simulink model "Vehicle_Model_2Track"  (R2021a)
settings: Solver=FixedStepDiscrete  StartTime=T0  StopTime=Tf  FixedStep=Ts  EnableMultiTasking=on
model workspace (MAT data in the model file):
  aKalman = Simulink.Parameter
  aKalman.DataType = 'auto'
  aKalman.Dimensions = [0 0]
  slipEnabler = Simulink.Parameter
  slipEnabler.DataType = 'auto'
  slipEnabler.Dimensions = [0 0]
values from neighbouring files (symbols this model uses):
  pacejkaParam = loadPacejkaParam()    [mainVehicleModel_2Track.m]
  vehicle_data = getVehicleDataStruct()    [mainVehicleModel_2Track.m]
  X0 = loadInitialConditions    [mainVehicleModel_2Track.m]
undefined symbols (not defined in the file or in its folder): DiscIntNeverNeededParam
libraries: simulink_extras x11
settings Model: Creator=Edoardo  LastModifiedBy=basemprince
settings SolverCC: AlgebraicLoopSolver=TrustRegion
settings DataIOCC: LimitDataPoints=on  SaveFormat=Array
settings OptimizationCC: DefaultParameterBehavior=Inlined  PassReuseOutputArgsAs=Individual arguments  MaxStackSize=64  EfficientTunableParamExpr=on
settings DebuggingCC: ReadBeforeWriteMsg=DisableAll  WriteAfterWriteMsg=DisableAll  WriteAfterReadMsg=DisableAll  MultiTaskDSMMsg=none  ParameterTunabilityLossMsg=error  PregeneratedLibrarySubsystemCodeDiagnostic=none  SFUnexpectedBacktrackingDiag=warning  SFNoUnconditionalDefaultTransitionDiag=warning  SFExecutionAtInitializationDiag=none  SFMachineParentedDataDiag=warning  ArithmeticOperatorsInVariantConditions=warning
settings HardwareCC: ProdBitPerInt=16  ProdBitPerPointer=16  ProdBitPerSizeT=16  ProdBitPerPtrDiffT=16  ProdLargestAtomicFloat=None  ProdWordSize=16  ProdHWDeviceType=STMicroelectronics->ST10/Super10
settings ModelReferenceCC: UpdateModelReferenceTargets=IfOutOfDate  PropagateSignalLabelsOutOfModel=off
settings SFSimCC: SFSimEcho=off  SimUseLocalCustomCode=off  MATLABDynamicMemAlloc=off  CustomCodeUndefinedFunction=UseInterfaceOnly
settings RTWCC: SystemTargetFile=ert.tlc  TemplateMakefile=ert_default_tmf  GenerateReport=on  RetainRTWFile=on  RTWUseLocalCustomCode=off  Toolchain=GNU Tools for ARM Embedded Processors  BuildConfiguration=Faster Runs  IncludeHyperlinkInReport=on  LaunchReport=on  GenerateTraceInfo=on  GenerateTraceReport=on  GenerateTraceReportSl=on  GenerateTraceReportSf=on  GenerateTraceReportEml=on
settings CodeAppCC: ForceParamTrailComments=on  IgnoreCustomStorageClasses=off  OperatorAnnotations=on  SimulinkDataObjDesc=on  SFDataObjDesc=on  InsertBlockDesc=on
settings ERTTargetCC: CodeReplacementLibrary=ARM Cortex-M (Optimized)  SupportVariableSizeSignals=on  RootIOFormat=Structure reference  ERTCustomFileTemplate=example_file_process.tlc
settings ConfigComp: CovMetricSettings=dw  CovSaveCumulativeToWorkspaceVar=on  CovSaveSingleToWorkspaceVar=on  CovExternalEMLEnable=off

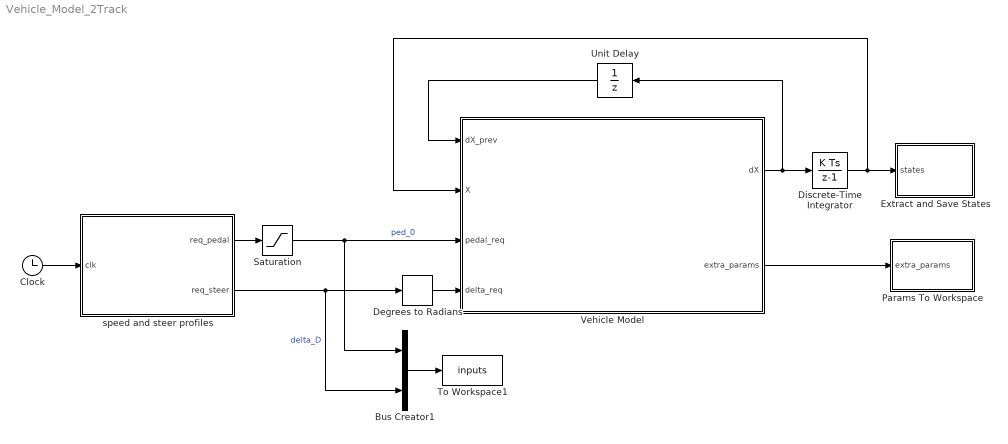
== system Vehicle_Model_2Track ==
  Bus Creator1 : BusCreator  Inputs=2
  Clock : Clock
  Degrees to Radians : simulink_extras/Transformations/Degrees to Radians
  Discrete-Time Integrator : DiscreteIntegrator  gainval=1  InitialCondition=X0  SampleTime=-1  ICPrevOutput=DiscIntNeverNeededParam  ICPrevScaledInput=DiscIntNeverNeededParam
  Extract and Save States : Subsystem
  Params To Workspace : Subsystem
  Saturation : Saturate  UpperLimit=1  LowerLimit=-1
  To Workspace1 : ToWorkspace  VariableName=inputs  SaveFormat=Timeseries  SampleTime=-1
  Unit Delay : UnitDelay  InitialCondition=zeros(size(X0))  SampleTime=-1  HasFrameUpgradeWarning=on
  Vehicle Model : MATLAB Function  TreatAsAtomicUnit=on
  speed and steer profiles : MATLAB Function  TreatAsAtomicUnit=on
  wires:
  Vehicle Model/2(extra_params) -> Params To Workspace/1(extra_params)
  Discrete-Time Integrator/1 -> Extract and Save States/1(states), Vehicle Model/2(X)
  Vehicle Model/1(dX) -> Unit Delay/1, Discrete-Time Integrator/1
  Bus Creator1/1 -> To Workspace1/1
  speed and steer profiles/2(req_steer) -> Bus Creator1/2, Degrees to Radians/1  "delta_D"
  Degrees to Radians/1 -> Vehicle Model/4(delta_req)
  speed and steer profiles/1(req_pedal) -> Saturation/1
  Clock/1 -> speed and steer profiles/1(clk)
  Saturation/1 -> Vehicle Model/3(pedal_req), Bus Creator1/1  "ped_0"
  Unit Delay/1 -> Vehicle Model/1(dX_prev)

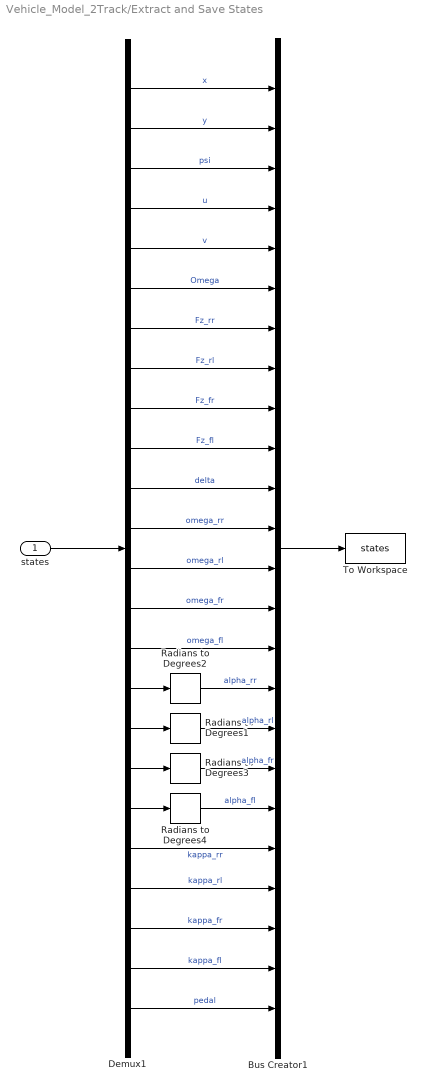
== system Vehicle_Model_2Track/Extract and Save States ==
  states : Inport
  Bus Creator1 : BusCreator  Inputs=24
  Demux1 : Demux  Outputs=24
  Radians to Degrees{1..4} (4 alike) : simulink_extras/Transformations/Radians to Degrees
  To Workspace : ToWorkspace  VariableName=states  SaveFormat=Timeseries  SampleTime=-1
  wires:
  Demux1/13 -> Bus Creator1/13  "omega_rl"
  Demux1/8 -> Bus Creator1/8  "Fz_rl"
  Demux1/23 -> Bus Creator1/23  "kappa_fl"
  Demux1/19 -> Radians to Degrees4/1
  states/1 -> Demux1/1
  Demux1/14 -> Bus Creator1/14  "omega_fr"
  Demux1/7 -> Bus Creator1/7  "Fz_rr"
  Demux1/15 -> Bus Creator1/15  "omega_fl"
  Demux1/3 -> Bus Creator1/3  "psi"
  Demux1/22 -> Bus Creator1/22  "kappa_fr"
  Demux1/4 -> Bus Creator1/4  "u"
  Demux1/6 -> Bus Creator1/6  "Omega"
  Demux1/11 -> Bus Creator1/11  "delta"
  Demux1/5 -> Bus Creator1/5  "v"
  Demux1/9 -> Bus Creator1/9  "Fz_fr"
  Demux1/21 -> Bus Creator1/21  "kappa_rl"
  Demux1/12 -> Bus Creator1/12  "omega_rr"
  Demux1/17 -> Radians to Degrees1/1
  Demux1/2 -> Bus Creator1/2  "y"
  Demux1/20 -> Bus Creator1/20  "kappa_rr"
  Demux1/10 -> Bus Creator1/10  "Fz_fl"
  Demux1/18 -> Radians to Degrees3/1
  Demux1/1 -> Bus Creator1/1  "x"
  Demux1/16 -> Radians to Degrees2/1
  Bus Creator1/1 -> To Workspace/1
  Radians to Degrees2/1 -> Bus Creator1/16  "alpha_rr"
  Radians to Degrees1/1 -> Bus Creator1/17  "alpha_rl"
  Radians to Degrees3/1 -> Bus Creator1/18  "alpha_fr"
  Radians to Degrees4/1 -> Bus Creator1/19  "alpha_fl"
  Demux1/24 -> Bus Creator1/24  "pedal"

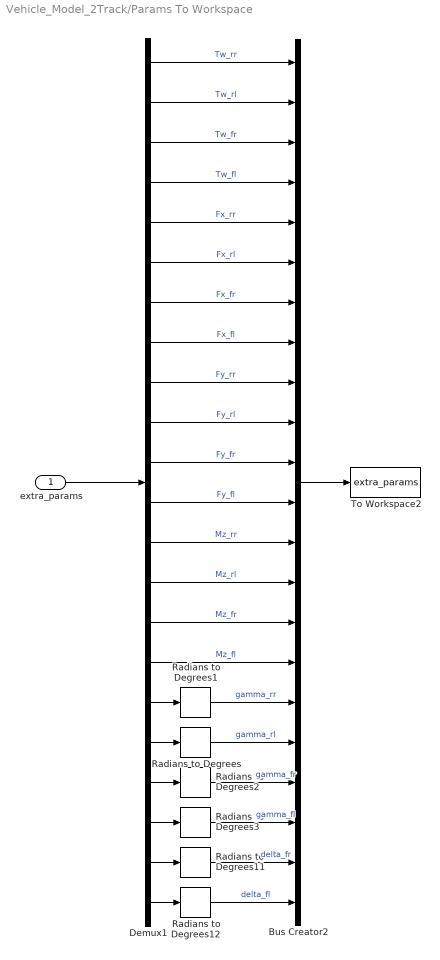
== system Vehicle_Model_2Track/Params To Workspace ==
  extra_params : Inport
  Bus Creator2 : BusCreator  Inputs=22
  Demux1 : Demux  Outputs=22
  Radians to Degrees{,1..3,11..12} (6 alike) : simulink_extras/Transformations/Radians to Degrees
  To Workspace2 : ToWorkspace  VariableName=extra_params  SaveFormat=Timeseries  SampleTime=-1
  wires:
  Demux1/17 -> Radians to Degrees1/1
  Demux1/3 -> Bus Creator2/3  "Tw_fr"
  Radians to Degrees3/1 -> Bus Creator2/20  "gamma_fl"
  Demux1/16 -> Bus Creator2/16  "Mz_fl"
  Radians to Degrees1/1 -> Bus Creator2/17  "gamma_rr"
  Radians to Degrees11/1 -> Bus Creator2/21  "delta_fr"
  Demux1/14 -> Bus Creator2/14  "Mz_rl"
  Demux1/4 -> Bus Creator2/4  "Tw_fl"
  Demux1/6 -> Bus Creator2/6  "Fx_rl"
  Demux1/8 -> Bus Creator2/8  "Fx_fl"
  Demux1/13 -> Bus Creator2/13  "Mz_rr"
  Demux1/7 -> Bus Creator2/7  "Fx_fr"
  Demux1/5 -> Bus Creator2/5  "Fx_rr"
  Demux1/9 -> Bus Creator2/9  "Fy_rr"
  Demux1/11 -> Bus Creator2/11  "Fy_fr"
  Demux1/15 -> Bus Creator2/15  "Mz_fr"
  Demux1/10 -> Bus Creator2/10  "Fy_rl"
  Radians to Degrees12/1 -> Bus Creator2/22  "delta_fl"
  Radians to Degrees2/1 -> Bus Creator2/19  "gamma_fr"
  extra_params/1 -> Demux1/1
  Demux1/12 -> Bus Creator2/12  "Fy_fl"
  Bus Creator2/1 -> To Workspace2/1
  Demux1/1 -> Bus Creator2/1  "Tw_rr"
  Demux1/2 -> Bus Creator2/2  "Tw_rl"
  Radians to Degrees/1 -> Bus Creator2/18  "gamma_rl"
  Demux1/18 -> Radians to Degrees/1
  Demux1/19 -> Radians to Degrees2/1
  Demux1/20 -> Radians to Degrees3/1
  Demux1/21 -> Radians to Degrees11/1
  Demux1/22 -> Radians to Degrees12/1

== matlab function Vehicle_Model_2Track/speed and steer profiles ==
  data: clk input; req_pedal output; req_steer output
function [req_pedal,req_steer] = pedal_steer_profiles(clk)

    % ----------------------------------------------------------------
    %% Function purpose: compute the desired pedal and steer profiles
    % ----------------------------------------------------------------
    
    % Requested pedal [-] in [-1,1] for this time step.
    % req_pedal > 0 means throttle
    % req_pedal < 0 means brake
    req_pedal = -0.5;
    
    % Requested steering angle [deg] at the steering wheel for this time step
    req_steer = 1*sin(2*pi*0.18*clk);

end

== matlab function Vehicle_Model_2Track/Vehicle Model ==
  settings: sampleTime=step_size
  data: dX_prev input; X input; dX output; extra_params output; pedal_req input; delta_req input; pacejkaParam parameter; vehicle_data parameter
function [dX,extra_params] = Vehicle_model(dX_prev,X,pedal_req,delta_req,pacejkaParam,vehicle_data)

% ----------------------------------------------------------------
%% Double Track Vehicle Model of Formula SAE electric vehicle (Chimera Evoluzione)
%  authors: Mattia Piccinini & Gastone Pietro Papini Rosati
%  email:  mattia.piccinini@unitn.it
%  date:   13/10/2020
% ----------------------------------------------------------------


% ----------------------------------------------------------------
%% INPUTS OF THE MODEL
% ----------------------------------------------------------------

% Model inputs are: 
%       - requested pedal (throttle if >0, brake if <0)
%       - requested steering angle at the steering wheel delta_req (in [rad])


% ----------------------------------------------------------------
%% OUTPUTS OF THE MODEL
% ----------------------------------------------------------------

% The outputs of the model are the derivatives of all vehicle states,
% collected in the dX vector, as well as some other useful extra parameters 
% to describe vehicle behavior, saved in the extra_params vector

% Empty output vectors are here initialized 
dX = zeros(24,1);  
extra_params = zeros(22,1);  


% ----------------------------------------------------------------
%% STATES OF THE MODEL
% ----------------------------------------------------------------

x         = X(1);       % [m] x-coord of the vehicle CoM
y         = X(2);       % [m] y-coord of the vehicle CoM
psi       = X(3);       % [rad] yaw angle
u         = X(4);       % [m/s] vehicle longitudinal speed
v         = X(5);       % [m/s] vehicle lateral speed
Omega     = X(6);       % [rad/s] yaw rate
Fz__rr    = X(7);       % [N] vertical force for the rear right wheel
Fz__rl    = X(8);       % [N] vertical force for the rear left wheel
Fz__fr    = X(9);       % [N] vertical force for the front right wheel
Fz__fl    = X(10);      % [N] vertical force for the front left wheel
delta     = X(11);      % [rad] steering angle (at the wheel)
omega__rr = X(12);      % [rad/s] rotational speed rear right wheel
omega__rl = X(13);      % [rad/s] rotational speed rear left wheel 
omega__fr = X(14);      % [rad/s] rotational speed front right wheel 
omega__fl = X(15);      % [rad/s] rotational speed front left wheel 
alpha__rr = X(16);      % [rad] side slip angle rear right wheel
alpha__rl = X(17);      % [rad] side slip angle rear left wheel
alpha__fr = X(18);      % [rad] side slip angle front right wheel
alpha__fl = X(19);      % [rad] side slip angle front left wheel
kappa__rr = X(20);      % [-] longitudinal slip rear right wheel
kappa__rl = X(21);      % [-] longitudinal slip rear left wheel
kappa__fr = X(22);      % [-] longitudinal slip front right wheel
kappa__fl = X(23);      % [-] longitudinal slip front left wheel
ped       = X(24);      % [-] pedal

% ----------------------------------------------------------------
%% AUXILIARY MODELS
% ----------------------------------------------------------------

% ----------------------
% MOTOR MODEL
% ----------------------
% Driving torques at the wheels
Tm_req = posPart(ped)*vehicle_data.motor.maxTorque;
Tw__rr_traction = MotorModel(Tm_req,omega__rr,vehicle_data);
Tw__rl_traction = MotorModel(Tm_req,omega__rl,vehicle_data);
 
% ----------------------
% BRAKE MODEL
% ----------------------
Tb_r_req = -negPart(ped)*vehicle_data.braking.totBrakeTorque*(1-vehicle_data.braking.brakeRatio);
Tb_f_req = -negPart(ped)*vehicle_data.braking.totBrakeTorque*vehicle_data.braking.brakeRatio;
% Rear wheels braking model
[Tw__rr_brake,Tw__rl_brake] = brakeModelRear(Tb_r_req,omega__rr,omega__rl,vehicle_data); 
% Front wheels braking model
[Tw__fr_brake,Tw__fl_brake] = brakeModelFront(Tb_f_req,omega__fr,omega__fl,vehicle_data);

% ----------------------
% WHEEL TORQUES
% ----------------------
% The total torque for each wheel is the algebraic sum of motor and brake torques
Tw__rr = Tw__rr_traction + Tw__rr_brake;
Tw__rl = Tw__rl_traction + Tw__rl_brake;
Tw__fr = Tw__fr_brake;
Tw__fl = Tw__fl_brake;

% ----------------------
% CAMBER MODEL
% ----------------------
[gamma__rr, gamma__rl, gamma__fr, gamma__fl] = camberModel(vehicle_data);

% ----------------------
% ACKERMANN STEERING MODEL
% ----------------------
% Compute steering angles for front wheels, with perfect Ackerman steering model
[delta__fr, delta__fl] = perfectAcker(delta,vehicle_data);

% ----------------------
% AERODYNAMIC MODEL
% ----------------------
% Aero drag, downforce at rear axle, downforce at front axle
[FAxc, FAz__r, FAz__f] = aeroModel(u,vehicle_data);
          
% ----------------------
% TIRE PACEJKA MODEL
% ----------------------
% Ensure symmetric behavior of left and right tires by calculating the
% forces and moments for left tires via a previous change of sign of the
% side slip alpha and the camber gamma
[Fx__rr,Fy__rr,AM__rr] = pacejka_model(kappa__rr,Fz__rr,alpha__rr,gamma__rr,pacejkaParam);
[Fx__rl,Fy__rl,AM__rl] = pacejka_model(kappa__rl,Fz__rl,-alpha__rl,-gamma__rl,pacejkaParam);
[Fx__fr,Fy__fr,AM__fr] = pacejka_model(kappa__fr,Fz__fr,alpha__fr,gamma__fr,pacejkaParam);
[Fx__fl,Fy__fl,AM__fl] = pacejka_model(kappa__fl,Fz__fl,-alpha__fl,-gamma__fl,pacejkaParam);
% Now perform a second change of sign in order to restore the correct operating conditions
Fy__rl = -Fy__rl; AM__rl = -AM__rl;
Fy__fl = -Fy__fl; AM__fl = -AM__fl;
Mz_tires.rr = AM__rr;  Mz_tires.rl = AM__rl;  Mz_tires.fr = AM__fr;  Mz_tires.fl = AM__fl;

% ----------------------
% VERTICAL TIRE FORCES MODEL
% ----------------------
% Compute vertical tire loads
u_dot = dX_prev(4);
VerticalForces = LoadTransferModel(Omega,u,u_dot,FAz__r,FAz__f,Mz_tires,vehicle_data);
Fz__rr__ss = VerticalForces.Fz_rr_ss;
Fz__rl__ss = VerticalForces.Fz_rl_ss;
Fz__fr__ss = VerticalForces.Fz_fr_ss;
Fz__fl__ss = VerticalForces.Fz_fl_ss;

% ----------------------
% AXLE FORCES
% ----------------------
Fx__r = Fx__rr + Fx__rl;  % ...
Fx__f = Fx__fl - sin(delta__fl)*Fy__fl + Fx__fr - sin(delta__fr) * Fy__fr;  % ...
Fy__r = Fy__rr + Fy__rl;  % ...
Fy__f = sin(delta__fl)* Fx__fl + Fy__fl + sin(delta__fr)*Fx__fr+ Fy__fr;  % ...
Delta__Fx__r = (Fx__rr-Fx__rl) / 2;  % ...
Delta__Fx__f = ((Fx__fr - sin(delta__fr)* Fy__fr) - (Fx__fl - sin(delta__fl)*Fy__fl))/2;  % ...

% ----------------------
% STEADY STATE SLIPS
% ----------------------
[kappa__rr__ss,kappa__rl__ss,kappa__fr__ss,kappa__fl__ss] = steadyStateLongSlips(omega__rr,omega__rl,omega__fr,omega__fl,Omega,u,delta__fr,delta__fl,vehicle_data);
[alpha__rr__ss,alpha__rl__ss,alpha__fr__ss,alpha__fl__ss] = steadyStateLatSlips(Omega,u,v,delta__fr,delta__fl,vehicle_data);


% ----------------------------------------------------------------
%% VEHICLE DATA
% ----------------------------------------------------------------
m      = vehicle_data.vehicle.m;
Lf     = vehicle_data.vehicle.Lf;
Lr     = vehicle_data.vehicle.Lr;
Wf     = vehicle_data.vehicle.Wf;
Wr     = vehicle_data.vehicle.Wr;
izz    = vehicle_data.vehicle.i_zz;
tau__N = vehicle_data.suspension.tau_N;
tau__D = vehicle_data.steering_system.tau_D;
tau__H = vehicle_data.steering_system.tau_H;
ly     = vehicle_data.vehicle.ly;
lx     = vehicle_data.vehicle.lx;
iwa__r = vehicle_data.rear_wheel.iwa_r;
iwa__f = vehicle_data.front_wheel.iwa_f;
Rr     = vehicle_data.rear_wheel.Rr;
Rf     = vehicle_data.front_wheel.Rf;
tau_ped = vehicle_data.motor.tau_ped;

% ----------------------------------------------------------------
%% VEHICLE MODEL DIFFERENTIAL EQUATIONS
% ----------------------------------------------------------------

% The following system of ODE is imported from Maple symbolic model

% Evolution of vehicle pose
x_dot        = u*cos(psi) - v*sin(psi);
y_dot        = v*cos(psi) + u*sin(psi);
psi_dot      = Omega;
% Newton equations
u_Dot        = (Omega * m * v - FAxc + Fx__f + Fx__r) / m;  % ...
v_Dot        = (-Omega * m * u + Fy__f + Fy__r) / m;  % ...
% Euler equation
Omega_Dot    = (Lf * Fy__f - Lr * Fy__r + Wf * Delta__Fx__f + Wr * Delta__Fx__r + AM__fl + AM__fr + AM__rl + AM__rr) / izz;  % ...
% Vertical loads first order dynamics
Fz_rr_Dot    = (-Fz__rr + Fz__rr__ss) / tau__N;  % ...
Fz_rl_Dot    = (-Fz__rl + Fz__rl__ss) / tau__N;  % ...
Fz_fr_Dot    = (-Fz__fr + Fz__fr__ss) / tau__N;  % ...
Fz_fl_Dot    = (-Fz__fl + Fz__fl__ss) / tau__N;  % ...
% Steering wheel first order dynamics
delta_Dot    = (-delta * tau__D + delta_req) / tau__D / tau__H;
% Side slip angle first order dynamics
alpha_rr_Dot = -(alpha__rr - alpha__rr__ss) * abs(u) / ly;  % ...
alpha_rl_Dot = -(alpha__rl - alpha__rl__ss) * abs(u) / ly;  % ...
alpha_fr_Dot = -(alpha__fr - alpha__fr__ss) * abs(u) / ly;  % ...
alpha_fl_Dot = -(alpha__fl - alpha__fl__ss) * abs(u) / ly;  % ...
% Longitudinal slip first order dynamics
kappa_rr_Dot = -abs(u) * (kappa__rr - kappa__rr__ss) / lx;  % ...
kappa_rl_Dot = -abs(u) * (kappa__rl - kappa__rl__ss) / lx;  % ...
kappa_fr_Dot = -abs(u) * (kappa__fr - kappa__fr__ss) / lx;  % ...
kappa_fl_Dot = -abs(u) * (kappa__fl - kappa__fl__ss) / lx;  % ...
% Wheel spin dynamics
omega_rr_Dot = (-Fx__rr * Rr + Tw__rr) / iwa__r;  % ...
omega_rl_Dot = (-Fx__rl * Rr + Tw__rl) / iwa__r;  % ...
omega_fr_Dot = (-Fx__fr * Rf + Tw__fr) / iwa__f;  % ...
omega_fl_Dot = (-Fx__fl * Rf + Tw__fl) / iwa__f;  % ...
% pedal dynamics
ped_Dot      = (pedal_req - ped) / tau_ped;

% Collect states derivatives in the dX vector
dX(1)  = x_dot;
dX(2)  = y_dot;
dX(3)  = psi_dot;
dX(4)  = u_Dot;
dX(5)  = v_Dot;
dX(6)  = Omega_Dot;
dX(7)  = Fz_rr_Dot;
dX(8)  = Fz_rl_Dot;
dX(9)  = Fz_fr_Dot;
dX(10) = Fz_fl_Dot;
dX(11) = delta_Dot;
dX(12) = omega_rr_Dot;
dX(13) = omega_rl_Dot;
dX(14) = omega_fr_Dot;
dX(15) = omega_fl_Dot;
dX(16) = alpha_rr_Dot;
dX(17) = alpha_rl_Dot;
dX(18) = alpha_fr_Dot;
dX(19) = alpha_fl_Dot;
dX(20) = kappa_rr_Dot;
dX(21) = kappa_rl_Dot;
dX(22) = kappa_fr_Dot;
dX(23) = kappa_fl_Dot;
dX(24) = ped_Dot;


% ----------------------------------------------------------------
%% SAVE USEFUL EXTRA PARAMETERS
% ----------------------------------------------------------------

extra_params(1)  = Tw__rr;
extra_params(2)  = Tw__rl;
extra_params(3)  = Tw__fr;
extra_params(4)  = Tw__fl;
extra_params(5)  = Fx__rr;
extra_params(6)  = Fx__rl;
extra_params(7)  = Fx__fr;
extra_params(8)  = Fx__fl;
extra_params(9)  = Fy__rr;
extra_params(10) = Fy__rl;
extra_params(11) = Fy__fr;
extra_params(12) = Fy__fl;
extra_params(13) = AM__rr;
extra_params(14) = AM__rl;
extra_params(15) = AM__fr;
extra_params(16) = AM__fl;
extra_params(17) = gamma__rr;
extra_params(18) = gamma__rl;
extra_params(19) = gamma__fr;
extra_params(20) = gamma__fl;
extra_params(21) = delta__fr;
extra_params(22) = delta__fl;

end
